simulink model "OpenLoop_old"  (R2023a)
settings: Solver=FixedStepAuto  StartTime=0.0  StopTime=29.4428  FixedStep=0.001  RelTol=1e-3  EnableMultiTasking=on
values from neighbouring files (symbols this model uses):
  t_control = t    [MAIN.m]    (also in MAIN_HW.m; step.mat = [0 0.10101010101 0.20202020202 0.30303030303 0.40404040404 0)
  ut = u    [MAIN.m]    (also in MAIN_HW.m; step.mat = [0 0 0 0 0 0 0 0 0 0 0.6 0.6 ... (100 elements, 1x100)])
  x0 = [-pi/2;0;0;0]    [MAIN.m]    (also in MAIN_HW.m; fitParams.m = [-pi/2; 0; 0; 0])
undefined symbols (not defined in the file or in its folder): DiscIntNeverNeededParam
settings Model: ExtModeTrigType=signal  ExtModeTrigDuration=60000  ExtModeTrigDirection=either  ExtModeTrigLevel=0.500000  Creator=colegiusto  LastModifiedBy=colegiusto
settings SolverCC: PositivePriorityOrder=on
settings OptimizationCC: BlockReduction=off  DefaultParameterBehavior=Inlined  BufferReuse=off
settings RTWCC: Description=QUARC Win64 Target Using Toolchain  SystemTargetFile=quarc_win64.tlc  Toolchain=QUARC win64 | nmake (64-bit Windows)  BuildConfiguration=Faster Runs
settings STFCustomTargetCC: TargetLangStandard=C89/C90 (ANSI)  SystemTargetFile=quarc_win64.tlc
settings GRTTargetCC: TargetLangStandard=C89/C90 (ANSI)  ParMdlRefBuildCompliant=off  CompOptLevelCompliant=off  CombineOutputUpdateFcns=off  MatFileLogging=off  CPPClassGenCompliant=off  GRTInterface=on  ExtMode=on  ExtModeMexFile=quarc_comm

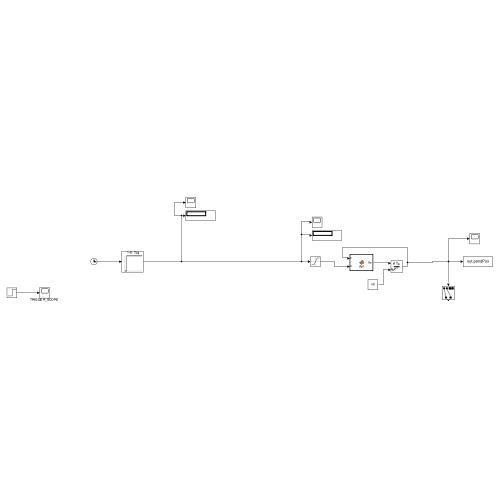
[thumbnail: Simulink's stored preview of the top-level diagram]
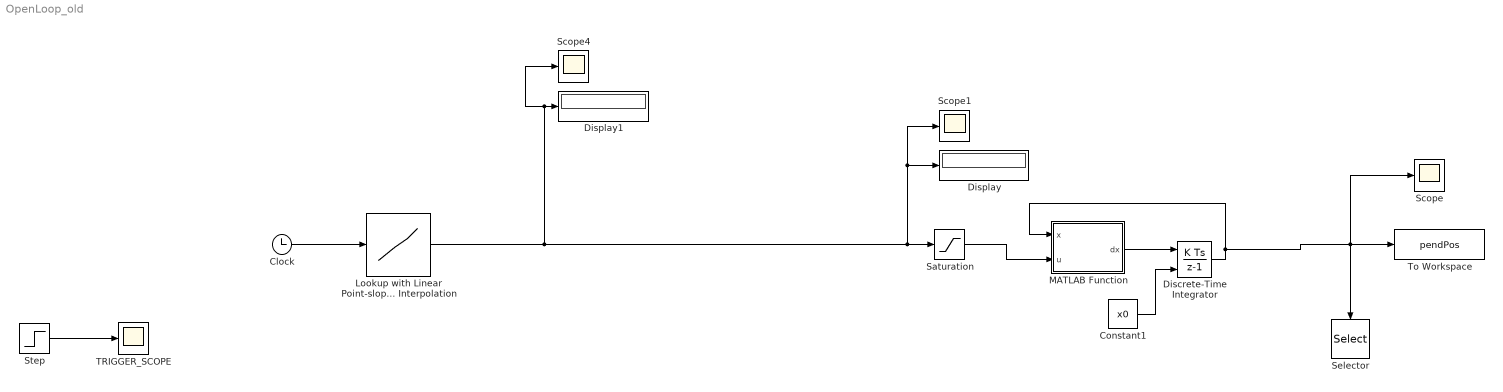
== system OpenLoop_old ==
  Clock : Clock
  Constant1 : Constant  Value=x0
  Discrete-Time Integrator : DiscreteIntegrator  InitialConditionSource=external  SampleTime=-1  ICPrevOutput=DiscIntNeverNeededParam  ICPrevScaledInput=DiscIntNeverNeededParam
  Display : Display
  Display1 : Display
  Lookup with Linear Point-slope Interpolation : Lookup_n-D  NumberOfTableDimensions=1  BreakpointsForDimension1=t_control  Table=ut  InternalRulePriority=Speed  RndMeth=Simplest
  MATLAB Function : MATLAB Function  TreatAsAtomicUnit=on
  Saturation : Saturate  UpperLimit=5  LowerLimit=-5
  Scope : Scope
  Scope1 : Scope
  Scope4 : Scope
  Selector : Selector  InputPortWidth=4  IndexOptions=Index vector (dialog)  Indices=[1,2]  OutputSizes=1
  Step : Step  Time=0.001  SampleTime=0
  TRIGGER_SCOPE : Scope
  To Workspace : ToWorkspace  VariableName=pendPos  SaveFormat=Structure With Time  SampleTime=-1
  wires:
  Step/1 -> TRIGGER_SCOPE/1
  Lookup with Linear Point-slope Interpolation/1 -> Saturation/1, Scope1/1, Display/1, Scope4/1, Display1/1
  Saturation/1 -> MATLAB Function/2(u)
  Constant1/1 -> Discrete-Time Integrator/2
  MATLAB Function/1(dx) -> Discrete-Time Integrator/1
  Discrete-Time Integrator/1 -> MATLAB Function/1(x), Selector/1, Scope/1, To Workspace/1
  Clock/1 -> Lookup with Linear Point-slope Interpolation/1

== matlab function OpenLoop_old/MATLAB Function ==
  data: x input; u input; dx output; p parameter
function dx = dyn(x,u,p)
    dx = dynamics(x,u,p);
end
